simulink model "izhikevichTest"  (R2020a)
settings: Solver=FixedStepAuto  StartTime=0.0  StopTime=1  FixedStep=0.001  RelTol=1e-3
libraries: simulink x2
settings Model: Creator=40129232  LastModifiedBy=40175607
settings DataIOCC: ReturnWorkspaceOutputs=off
settings OptimizationCC: LifeSpan=inf
settings DebuggingCC: SFExecutionAtInitializationDiag=none  ArithmeticOperatorsInVariantConditions=warning
settings SFSimCC: SimUseLocalCustomCode=off  CustomCodeUndefinedFunction=UseInterfaceOnly
settings RTWCC: RTWUseLocalCustomCode=off
settings CodeAppCC: StateflowObjectComments=on

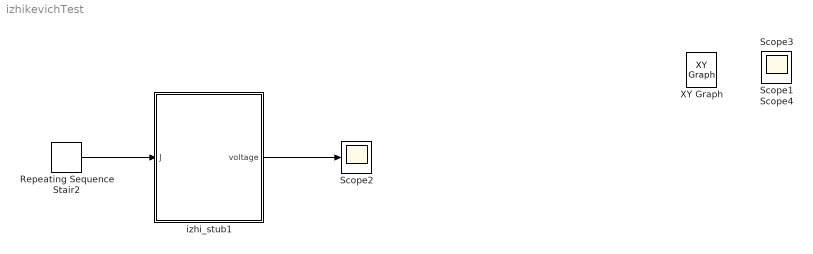
== system izhikevichTest ==
  Repeating Sequence Stair2 : simulink/Sources/Repeating Sequence Stair  OutValues=[40.37, 52.35, 62.17, 70.19, 76.75].'  tsamp=-1  OutMin=[]  OutMax=[]  OutDataTypeStr=double  OutputDataTypeScalingMode=double  OutDataType=fixdt(0,8)  ConRadixGroup=Best Precision: Vector-wise  OutScaling=2^-12
  Scope{1..4} (4 alike) : Scope
  izhi_stub1 : Subsystem
  XY Graph : simulink/Sinks/XY Graph  IOType=viewer  xmin=-1  xmax=1  ymin=-1  ymax=1  st=-1
  wires:
  izhi_stub1/1(voltage) -> Scope2/1
  Repeating Sequence Stair2/1 -> izhi_stub1/1(J)

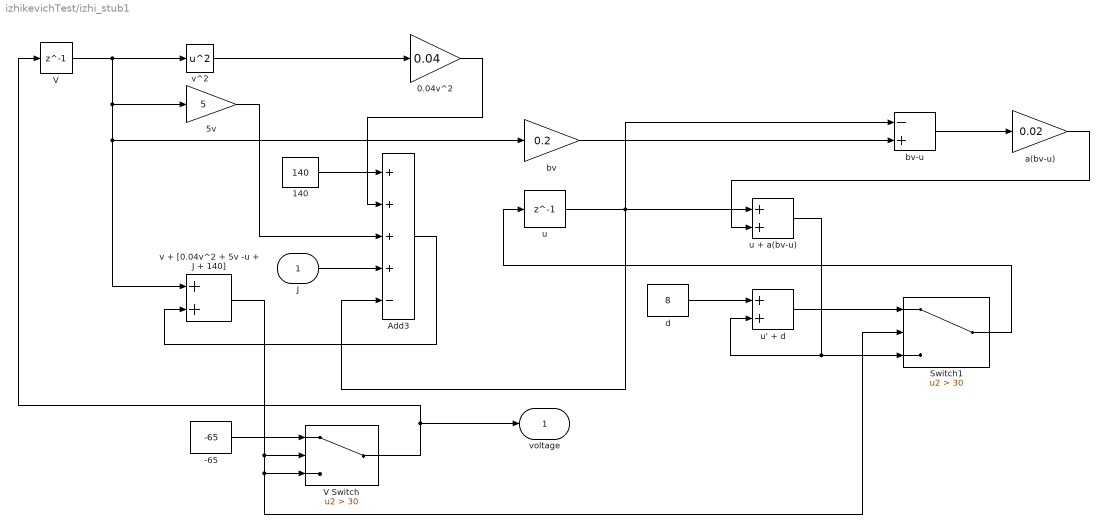
== system izhikevichTest/izhi_stub1 ==
  J : Inport
  -65 : Constant  Value=-65
  0.04v^2 : Gain  Gain=0.04
  140 : Constant  Value=140
  5v : Gain  Gain=5
  Add3 : Sum  Inputs=++++-
  Switch1 : Switch  Criteria=u2 > Threshold  Threshold=30
  V : Delay  DelayLength=1  InitialCondition=-65
  V Switch : Switch  Criteria=u2 > Threshold  Threshold=30
  a(bv-u) : Gain  Gain=0.02
  bv : Gain  Gain=0.2
  bv-u : Sum  Inputs=-+
  d : Constant  Value=8
  u : Delay  DelayLength=1  InitialCondition=0
  u + a(bv-u) : Sum
  u' + d : Sum
  v + [0.04v^2 + 5v -u + J + 140] : Sum
  v^2 : Math  Operator=square  SaturateOnIntegerOverflow=on
  voltage : Outport  VectorParamsAs1DForOutWhenUnconnected=off
  wires:
  5v/1 -> Add3/3
  0.04v^2/1 -> Add3/2
  Add3/1 -> v + [0.04v^2 + 5v -u + J + 140]/2
  V/1 -> v^2/1, v + [0.04v^2 + 5v -u + J + 140]/1, bv/1, 5v/1
  140/1 -> Add3/1
  u/1 -> Add3/5, bv-u/1, u + a(bv-u)/1
  v^2/1 -> 0.04v^2/1
  J/1 -> Add3/4
  bv/1 -> bv-u/2
  bv-u/1 -> a(bv-u)/1
  d/1 -> u' + d/1
  Switch1/1 -> u/1
  a(bv-u)/1 -> u + a(bv-u)/2
  V Switch/1 -> V/1, voltage/1
  -65/1 -> V Switch/1
  v + [0.04v^2 + 5v -u + J + 140]/1 -> Switch1/2, V Switch/3, V Switch/2
  u' + d/1 -> Switch1/1
  u + a(bv-u)/1 -> u' + d/2, Switch1/3
